simulink model "Lead_Lag_Controller"  (R2025b)
settings: Solver=VariableStepAuto  StartTime=0.0  StopTime=0.1  RelTol=1e-3
values from neighbouring files (symbols this model uses):
  den = [L*C/(1-D)^2, L/(R*(1-D)^2), 1]    [system_parameters.m]
  num = [Vin/(1-D)^2 * (-L/(R*(1-D)^2)), Vin/(1-D)^2]    [system_parameters.m]
settings Model: Creator=Seyma  LastModifiedBy=Seyma

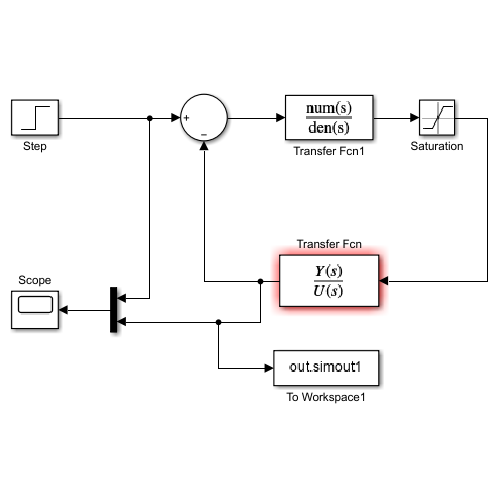
[thumbnail: Simulink's stored preview of the top-level diagram]
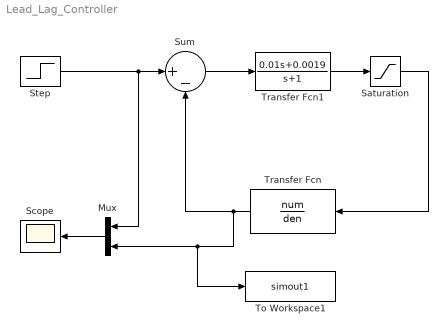
== system Lead_Lag_Controller ==
  Mux : Mux  Inputs=2
  Saturation : Saturate  UpperLimit=0.9  LowerLimit=0.1
  Scope : Scope
      settings: ActiveDisplayYMinimum=-10.817693100707595  ActiveDisplayYMaximum=47.999841108707038
  Step : Step  Time=0  After=24  SampleTime=0
  Sum : Sum  Inputs=|+-
  To Workspace1 : ToWorkspace  VariableName=simout1  SaveFormat=Timeseries  SampleTime=-1
  Transfer Fcn : TransferFcn  Numerator=num  Denominator=den
  Transfer Fcn1 : TransferFcn  Numerator=[0.01 0.0019]  Denominator=[1 1]
  wires:
  Mux/1 -> Scope/1
  Transfer Fcn/1 -> Sum/2, To Workspace1/1, Mux/2
  Step/1 -> Sum/1, Mux/1
  Saturation/1 -> Transfer Fcn/1
  Transfer Fcn1/1 -> Saturation/1
  Sum/1 -> Transfer Fcn1/1
